simulink model "Regulator_PI"  (R2022a)
settings: Solver=VariableStepAuto  StartTime=0.0  StopTime=10.0  RelTol=1e-3
values from neighbouring files (symbols this model uses):
  k_i = 0.37    [Regulatory_P_oraz_PI.m]
  k_p = 0.1    [Regulatory_P_oraz_PI.m]
settings Model: Creator=L13-6  LastModifiedBy=Filip
settings SolverCC: AlgebraicLoopSolver=TrustRegion
settings DataIOCC: ReturnWorkspaceOutputs=off
settings DebuggingCC: UnconnectedInputMsg=warning  UnconnectedOutputMsg=warning  UnconnectedLineMsg=warning  SFMachineParentedDataDiag=warning  ArithmeticOperatorsInVariantConditions=warning
settings SFSimCC: SimUseLocalCustomCode=off  CustomCodeUndefinedFunction=UseInterfaceOnly
settings RTWCC: RTWUseLocalCustomCode=off

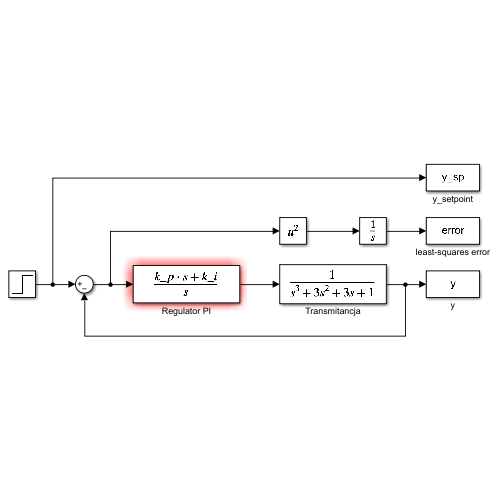
[thumbnail: Simulink's stored preview of the top-level diagram]
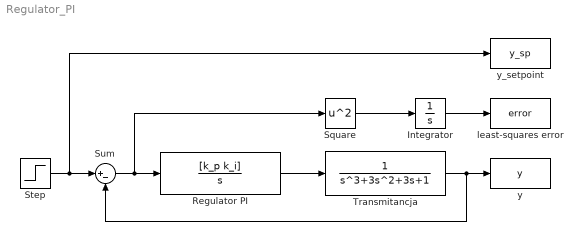
== system Regulator_PI ==
  Integrator : Integrator
  Regulator PI : TransferFcn  Numerator=[k_p k_i]  Denominator=[1 0]
  Square : Math  Operator=square  SignedPower=on  RndMeth=Zero
  Step : Step  SampleTime=0
  Sum : Sum  Inputs=|+-
  Transmitancja : TransferFcn  Denominator=[1 3 3 1]
  least-squares error : ToWorkspace  VariableName=error  SampleTime=-1
  y : ToWorkspace  VariableName=y  SampleTime=-1
  y_setpoint : ToWorkspace  VariableName=y_sp  SampleTime=-1
  wires:
  Integrator/1 -> least-squares error/1
  Step/1 -> Sum/1, y_setpoint/1
  Square/1 -> Integrator/1
  Sum/1 -> Regulator PI/1, Square/1
  Transmitancja/1 -> Sum/2, y/1
  Regulator PI/1 -> Transmitancja/1
